simulink model "practica2a"  (R2022a)
settings: Solver=FixedStepAuto  StartTime=0.0  StopTime=10.0  RelTol=1e-3  EnableMultiTasking=on
undefined symbols (not defined in the file): P, t_sim, TP
libraries: legoev3lib x6, simulink x1
settings Model: ExtModeTrigDuration=2  Creator=alumnopr09  LastModifiedBy=Sersa
settings SolverCC: AlgebraicLoopSolver=TrustRegion  PositivePriorityOrder=on
settings OptimizationCC: EnhancedBackFolding=on  PassReuseOutputArgsAs=Individual arguments  ZeroExternalMemoryAtStartup=off  ZeroInternalMemoryAtStartup=off  MaxStackSize=64  OptimizeBlockOrder=speed  DifferentSizesBufferReuse=on  OptimizationCustomize=off  EfficientTunableParamExpr=on
settings DebuggingCC: ParameterTunabilityLossMsg=error  UnconnectedInputMsg=warning  UnconnectedOutputMsg=warning  UnconnectedLineMsg=warning  SFMachineParentedDataDiag=warning
settings HardwareCC: ProdBitPerPointer=32  ProdBitPerSizeT=32  ProdBitPerPtrDiffT=32  ProdLargestAtomicInteger=Long  ProdWordSize=32  ProdHWDeviceType=ARM Compatible->ARM 9
settings SFSimCC: MATLABDynamicMemAlloc=off
settings RTWCC: SystemTargetFile=ert.tlc  HardwareBoard=LEGO MINDSTORMS EV3  TLCOptions="-aInlineSetEventsForThisBaseRateFcn=TLC_FALSE -aSuppressMultiTaskScheduler=TLC_FALSE  -aRateBasedStepFcn=0"  TemplateMakefile=ert_default_tmf  GenerateReport=on  Toolchain=Sourcery G++ Lite v2009q3  IncludeHyperlinkInReport=on  LaunchReport=on  GenerateTraceInfo=on  GenerateTraceReport=on  GenerateTraceReportSl=on  GenerateTraceReportSf=on  GenerateTraceReportEml=on
settings CodeAppCC: ForceParamTrailComments=on  IgnoreCustomStorageClasses=off  OperatorAnnotations=on  SimulinkDataObjDesc=on  SFDataObjDesc=on  InsertBlockDesc=on
settings ERTTargetCC: SupportContinuousTime=on  SupportVariableSizeSignals=on

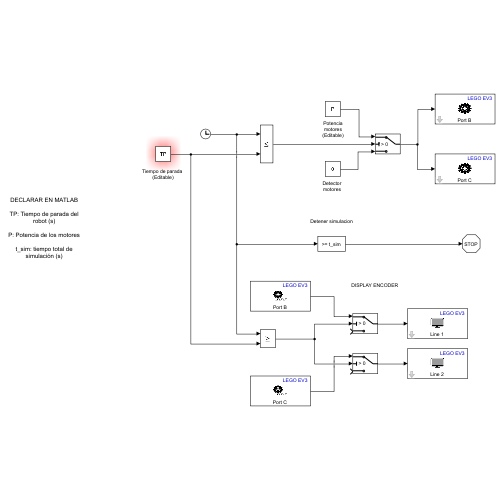
[thumbnail: Simulink's stored preview of the top-level diagram]
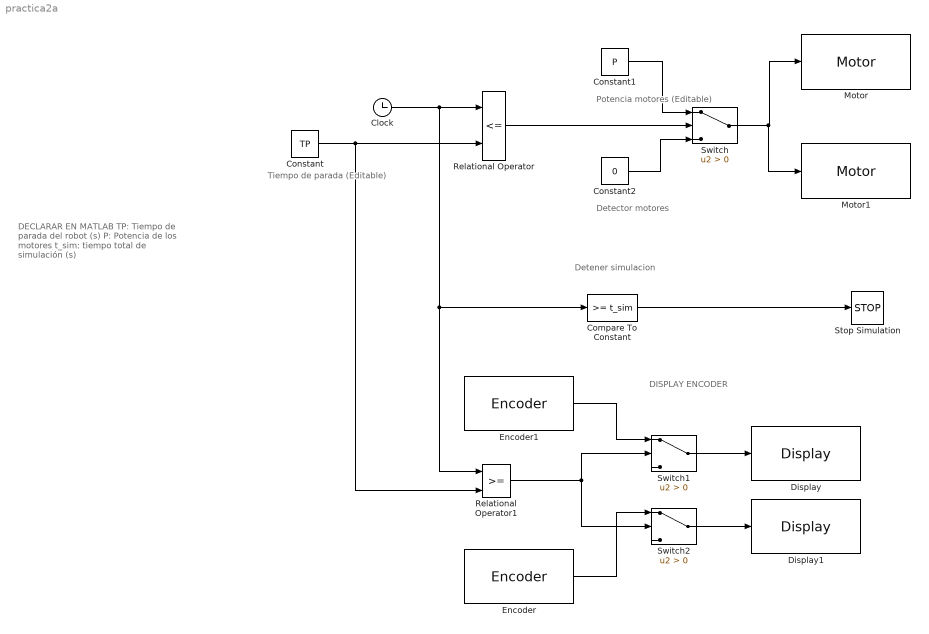
== system practica2a ==
  note: DECLARAR EN MATLAB
      |
      | TP: Tiempo de parada del robot (s)
      |
      | P: Potencia de los motores
      |
      | t_sim: tiempo total de simulación (s)
  note: DISPLAY ENCODER
  note: Detener simulacion
  note: Tiempo de parada
      | (Editable)
  note: Potencia
      | motores
      | (Editable)
  note: Detector
      | motores
  Clock : Clock
  Compare To Constant : simulink/Logic and Bit Operations/Compare To Constant  relop=>=  const=t_sim  OutDataTypeStr=boolean
  Constant : Constant  Value=TP
  Constant1 : Constant  Value=P
  Constant2 : Constant  Value=0
  Display : legoev3lib/Display  slcdLine=1  slcdFormat=Decimal
      settings: SourceProductBaseCode=LEGOEV3
  Display1 : legoev3lib/Display  slcdLine=2  slcdFormat=Decimal
      settings: SourceProductBaseCode=LEGOEV3
  Encoder : legoev3lib/Encoder  portNumber=C  opMode=No reset  sampleTime=0.1
      settings: SourceProductBaseCode=LEGOEV3
  Encoder1 : legoev3lib/Encoder  portNumber=B  opMode=No reset  sampleTime=0.1
      settings: SourceProductBaseCode=LEGOEV3
  Motor : legoev3lib/Motor  sportNumber=B  sstopAction=Brake
  Motor1 : legoev3lib/Motor  sportNumber=C  sstopAction=Brake
  Relational Operator : RelationalOperator  Operator=<=  OutDataTypeStr=boolean  RndMeth=Simplest  InputSameDT=off
  Relational Operator1 : RelationalOperator  OutDataTypeStr=boolean  RndMeth=Simplest  InputSameDT=off
  Stop Simulation : Stop
  Switch : Switch  Criteria=u2 > Threshold  SaturateOnIntegerOverflow=off  InputSameDT=off
  Switch1 : Switch  Criteria=u2 > Threshold  SaturateOnIntegerOverflow=off  InputSameDT=off
  Switch2 : Switch  Criteria=u2 > Threshold  SaturateOnIntegerOverflow=off  InputSameDT=off
  wires:
  Clock/1 -> Compare To Constant/1, Relational Operator1/1, Relational Operator/1
  Constant/1 -> Relational Operator1/2, Relational Operator/2
  Relational Operator/1 -> Switch/2
  Constant1/1 -> Switch/1
  Constant2/1 -> Switch/3
  Switch/1 -> Motor1/1, Motor/1
  Compare To Constant/1 -> Stop Simulation/1
  Relational Operator1/1 -> Switch2/2, Switch1/2
  Encoder1/1 -> Switch1/1
  Encoder/1 -> Switch2/1
  Switch2/1 -> Display1/1
  Switch1/1 -> Display/1
